simulink model "Furuta_Pendulum_Pole_Placement_With_Full_Order_Estimator"  (R2018a)
settings: Solver=ode45  StartTime=0.0  StopTime=10  RelTol=1e-3  EnableMultiTasking=on
values from neighbouring files (symbols this model uses):
  Ac = [0 1 0 0 ... (first row only)    [BasicModelParameters.m]    (also in ControllerDesign_REV0.m; FurutaPendulum.m = [0 1 0 0; 0 0 -a23 0; 0 0 0 1; 0 0 a43 0]; InvertedPendulumStepResponse.m)
  Bc = transpose([0 b21 0 -b41])    [BasicModelParameters.m]    (also in ControllerDesign_REV0.m; FurutaPendulum.m = [0; b21; 0; -b41]; InvertedPendulumStepResponse.m)
  Cc = [1 0 0 0 ... (first row only)    [BasicModelParameters.m]    (also in ControllerDesign_REV0.m; FurutaPendulum.m = [1 0 0 0; 0 0 1 0]; InvertedPendulumStepResponse.m)
  Dc = [0 ... (first row only)    [BasicModelParameters.m]    (also in ControllerDesign_REV0.m; FurutaPendulum.m = [0; 0]; InvertedPendulumStepResponse.m)
  K_s = place(Ac,Bc,Pcld_s)    [FurutaPendulum.m]
  Kdc_s = evalfr(Hcl_s(1),0)    [FurutaPendulum.m]
  L_s = place(Ac',Cc',Pestd_s)'    [FurutaPendulum.m]
  T = 0.01    [FurutaPendulum.m]
settings Model: Creator=James Carroll  LastModifiedBy=Jack
settings DataIOCC: LimitDataPoints=on  SaveFormat=Array  SignalLoggingSaveFormat=ModelDataLogs
settings OptimizationCC: ExpressionDepthLimit=2147483647  InitFltsAndDblsToZero=on  LifeSpan=inf
settings DebuggingCC: SolverPrmCheckMsg=warning  StateNameClashWarn=warning  SFUnexpectedBacktrackingDiag=warning  SFNoUnconditionalDefaultTransitionDiag=warning  SFExecutionAtInitializationDiag=none
settings HardwareCC: ProdBitPerPointer=32  ProdBitPerSizeT=32  ProdBitPerPtrDiffT=32  ProdLargestAtomicFloat=None  ProdIntDivRoundTo=Undefined  ProdEndianess=Unspecified  ProdWordSize=32  ProdHWDeviceType=32-bit Generic
settings ModelReferenceCC: PropagateSignalLabelsOutOfModel=off
settings CodeAppCC: StateflowObjectComments=on
settings GRTTargetCC: TargetLangStandard=C89/C90 (ANSI)  CombineOutputUpdateFcns=off  GRTInterface=on
settings ConfigComp: CovMetricSettings=dw  CovHtmlReporting=on  CovSaveCumulativeToWorkspaceVar=on  CovSaveSingleToWorkspaceVar=on  CovExternalEMLEnable=off

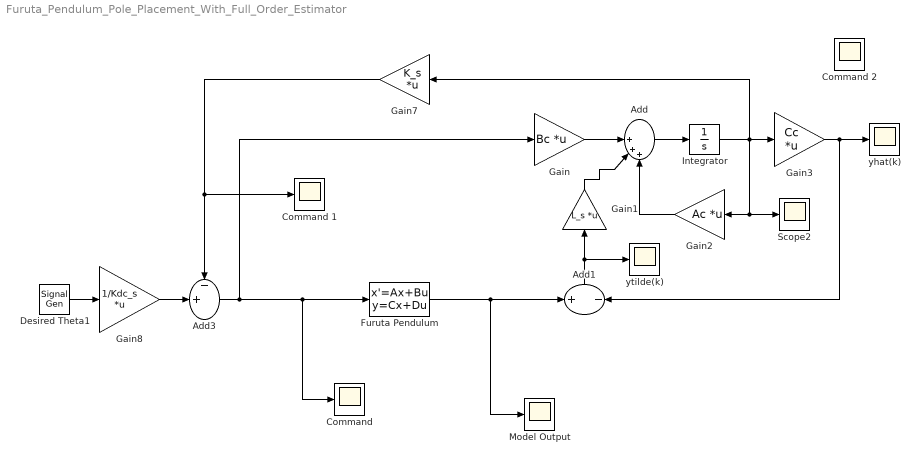
== system Furuta_Pendulum_Pole_Placement_With_Full_Order_Estimator ==
  " Model Output" : Scope
  Add : Sum  Inputs=||+++
  Add1 : Sum  Inputs=+-
  Add3 : Sum  Inputs=-+|
  "Command " : Scope
  Command 1 : Scope
  Command 2 : Scope
  Desired Theta1 : SignalGenerator  Amplitude=pi/4  Frequency=.1
  Furuta Pendulum : StateSpace  A=Ac  B=Bc  C=Cc  D=Dc  InitialCondition=[0; 0; 0.05; 0]  ContinuousStateAttributes='Theta'
  Gain : Gain  Gain=Bc  Multiplication=Matrix(K*u)
  Gain1 : Gain  Gain=L_s  Multiplication=Matrix(K*u)
  Gain2 : Gain  Gain=Ac  Multiplication=Matrix(K*u)
  Gain3 : Gain  Gain=Cc  Multiplication=Matrix(K*u)
  Gain7 : Gain  Gain=K_s  Multiplication=Matrix(K*u)
  Gain8 : Gain  Gain=1/Kdc_s  Multiplication=Matrix(K*u)  SampleTime=T
  Integrator : Integrator
  Scope2 : Scope
  yhat(k) : Scope
  ytilde(k) : Scope
  wires:
  Gain/1 -> Add/1
  Furuta Pendulum/1 -> " Model Output"/1, Add1/1
  Add1/1 -> Gain1/1, ytilde(k)/1
  Gain1/1 -> Add/2
  Add/1 -> Integrator/1
  Integrator/1 -> Gain3/1, Gain2/1, Scope2/1, Gain7/1
  Gain2/1 -> Add/3
  Gain3/1 -> yhat(k)/1, Add1/2
  Desired Theta1/1 -> Gain8/1
  Gain8/1 -> Add3/2
  Add3/1 -> "Command "/1, Furuta Pendulum/1, Gain/1
  Gain7/1 -> Command 1/1, Add3/1
